simulink model "lateral_autopilot_full"  (R2016b)
settings: Solver=VariableStepAuto  StartTime=0.0  StopTime=t_end  RelTol=1e-3
values from neighbouring files (symbols this model uses):
  A = [ -0.322 0.052 0.028 -1.12 ... (first row only)    [parameters_P3.m]    (also in parameters_longitudal_autopilot.m = [ -0.322 0.052 0.028 -1.12 0.002)
  B = [ 0.002 0 -0.65 -0.02]'    [parameters_P3.m]    (also in parameters_longitudal_autopilot.m = [ 0 0 0 0 10]')
  C = [0 0 1 0 ... (first row only)    [parameters_P3.m]    (also in parameters_longitudal_autopilot.m = [0 0 0 1 0)
  d = 2*deg2rad    [run_task_2e.m]    (also in run_task_2f.m; run_task_2g.m = 30*deg2rad)
  D = [0 0 0]'    [parameters_P3.m]    (also in parameters_longitudal_autopilot.m = [0 0 0 0]')
  delta_a_max = 25*deg2rad    (= 0.436332312999)    [parameters_P3.m]    (also in parameters_longitudal_autopilot.m)
  g = 9.81    [parameters_P3.m]    (also in parameters_longitudal_autopilot.m)
  k_d_phi = (2*zeta_phi*omega_n_phi - a_phi_1) / a_phi_2    [parameters_P3.m]    (also in parameters_longitudal_autopilot.m)
  k_i_chi = omega_n_chi^2*V_g/g    [parameters_P3.m]    (also in parameters_longitudal_autopilot.m; regulation_parameters_2_2.m)
  k_i_phi = 0    [parameters_P3.m]    (also in parameters_longitudal_autopilot.m)
  k_p_chi = 2*zeta_chi*omega_n_chi*V_g/g    [parameters_P3.m]    (also in parameters_longitudal_autopilot.m; regulation_parameters_2_2.m)
  k_p_phi = sign(a_phi_2)*delta_a_max /e_phi_max    [parameters_P3.m]    (also in parameters_longitudal_autopilot.m)
  V_g = 637/3.6    (= 176.944444444)    [parameters_P3.m]    (also in parameters_longitudal_autopilot.m)
settings Model: Creator=EllaLovise  LastModifiedBy=Alexandra

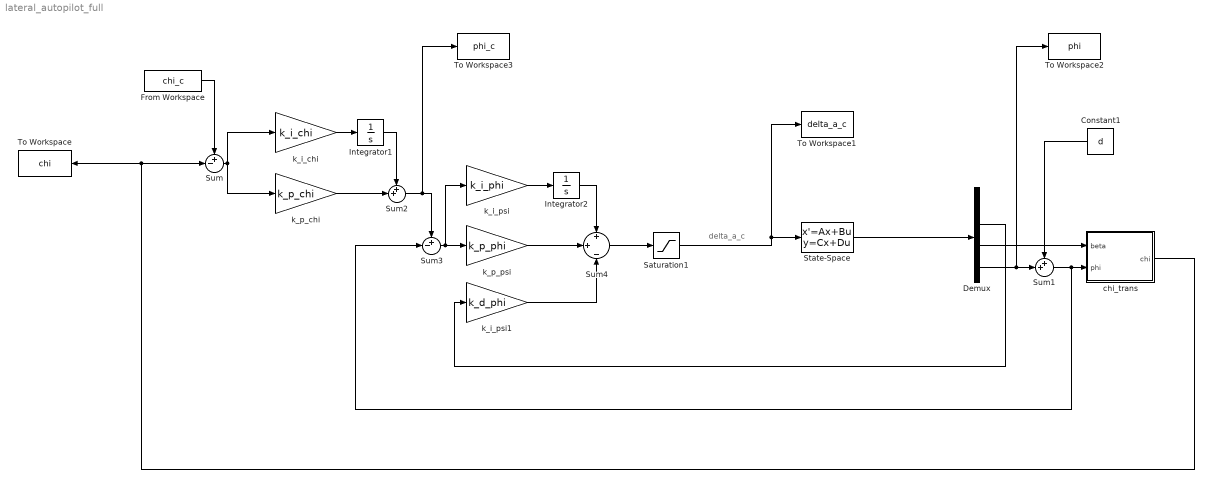
== system lateral_autopilot_full ==
  note: delta_a_c
  Constant1 : Constant  Value=d
  Demux : Demux
  From Workspace : FromWorkspace  VariableName=chi_c  OutputAfterFinalValue=Holding final value
  Integrator1 : Integrator
  Integrator2 : Integrator
  Saturation1 : Saturate  UpperLimit=delta_a_max  LowerLimit=-1*delta_a_max
  State-Space : StateSpace  A=A  B=B  C=C  D=D  X0=0
  Sum : Sum  Inputs=+-|
  Sum1 : Sum  Inputs=++|
  Sum2 : Sum  Inputs=++|
  Sum3 : Sum  Inputs=+-|
  Sum4 : Sum  Inputs=+|+|-
  To Workspace : ToWorkspace  VariableName=chi  SaveFormat=Structure With Time  SampleTime=-1
  To Workspace1 : ToWorkspace  VariableName=delta_a_c  SaveFormat=Structure With Time  SampleTime=-1
  To Workspace2 : ToWorkspace  VariableName=phi  SaveFormat=Structure With Time  SampleTime=-1
  To Workspace3 : ToWorkspace  VariableName=phi_c  SaveFormat=Structure With Time  SampleTime=-1
  chi_trans : Subsystem
  k_i_chi : Gain  Gain=k_i_chi
  k_i_psi : Gain  Gain=k_i_phi
  k_i_psi1 : Gain  Gain=k_d_phi
  k_p_chi : Gain  Gain=k_p_chi
  k_p_psi : Gain  Gain=k_p_phi
  wires:
  From Workspace/1 -> Sum/1
  Sum/1 -> k_i_chi/1, k_p_chi/1
  k_p_chi/1 -> Sum2/2
  Sum2/1 -> To Workspace3/1, Sum3/1
  Sum3/1 -> k_i_psi/1, k_p_psi/1
  k_i_psi/1 -> Integrator2/1
  chi_trans/1(chi) -> Sum/2, To Workspace/1
  k_i_chi/1 -> Integrator1/1
  Integrator1/1 -> Sum2/1
  Integrator2/1 -> Sum4/1
  k_p_psi/1 -> Sum4/2
  k_i_psi1/1 -> Sum4/3
  Demux/4 -> To Workspace2/1, Sum1/2
  Demux/3 -> chi_trans/1(beta)
  Demux/2 -> k_i_psi1/1
  Saturation1/1 -> To Workspace1/1, State-Space/1
  Sum4/1 -> Saturation1/1
  State-Space/1 -> Demux/1
  Constant1/1 -> Sum1/1
  Sum1/1 -> Sum3/2, chi_trans/2(phi)

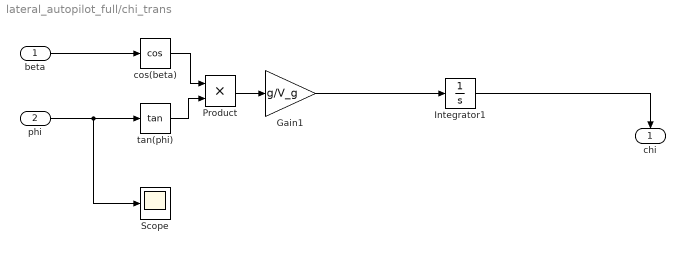
== system lateral_autopilot_full/chi_trans ==
  beta : Inport
  phi : Inport  Port=2
  Gain1 : Gain  Gain=g/V_g
  Integrator1 : Integrator
  Product : Product
  Scope : Scope
  cos(beta) : Trigonometry  Operator=cos
  tan(phi) : Trigonometry  Operator=tan
  chi : Outport
  wires:
  phi/1 -> Scope/1, tan(phi)/1
  Integrator1/1 -> chi/1
  beta/1 -> cos(beta)/1
  tan(phi)/1 -> Product/2
  Product/1 -> Gain1/1
  cos(beta)/1 -> Product/1
  Gain1/1 -> Integrator1/1
